simulink model "w2p4"  (R2020b)
settings: Solver=VariableStepAuto  StartTime=0.0  StopTime=10.0  RelTol=1e-3
model workspace (MAT data in the model file):
  J = Simulink.Parameter
  J.Value = 0.01
  J.DataType = 'auto'
  J.Dimensions = [1 1]
  K = Simulink.Parameter
  K.Value = 0.01
  K.DataType = 'auto'
  K.Dimensions = [1 1]
  Kd = Simulink.Parameter
  Kd.Value = 10
  Kd.DataType = 'auto'
  Kd.Dimensions = [1 1]
  Ki = Simulink.Parameter
  Ki.Value = 350
  Ki.DataType = 'auto'
  Ki.Dimensions = [1 1]
  Kp = 300
  L = Simulink.Parameter
  L.Value = 0.5
  L.DataType = 'auto'
  L.Dimensions = [1 1]
  R = Simulink.Parameter
  R.Value = 1
  R.DataType = 'auto'
  R.Dimensions = [1 1]
  b = 0.1
settings Model: Creator=Dell  LastModifiedBy=Dell

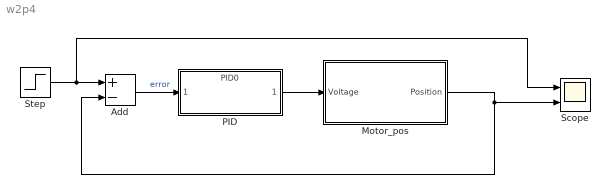
== system w2p4 ==
  Add : Sum  Inputs=+-
  Motor_pos : Subsystem
  PID : ModelReference  ModelNameDialog=PID0  SimulationMode=Normal  ModelReferenceVersion=1.3
  Scope : Scope  NumInputPorts=2
  Step : Step  SampleTime=0
  wires:
  Motor_pos/1(Position) -> Add/2, Scope/2
  PID/1 -> Motor_pos/1(Voltage)
  Step/1 -> Scope/1, Add/1
  Add/1 -> PID/1  "error"

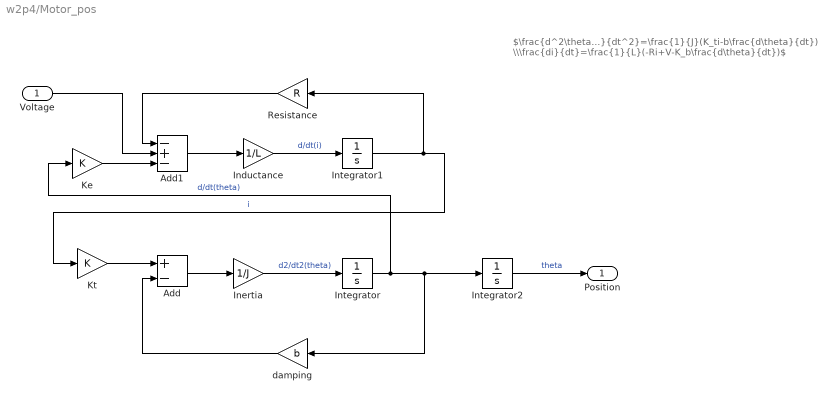
== system w2p4/Motor_pos ==
  note: $\frac{d^2\theta}{dt^2}=\frac{1}{J}(K_ti-b\frac{d\theta}{dt}) \\\frac{di}{dt}=\frac{1}{L}(-Ri+V-K_b\frac{d\theta}{dt})$
  Voltage : Inport
  Add : Sum  Inputs=+-
  Add1 : Sum  Inputs=-+-
  Inductance : Gain  Gain=1/L
  Inertia : Gain  Gain=1/J
  Integrator : Integrator
  Integrator1 : Integrator
  Integrator2 : Integrator
  Ke : Gain  Gain=K
  Kt : Gain  Gain=K
  Resistance : Gain  Gain=R
  damping : Gain  Gain=b
  Position : Outport
  wires:
  damping/1 -> Add/2
  Resistance/1 -> Add1/1
  Kt/1 -> Add/1
  Inductance/1 -> Integrator1/1  "d/dt(i)"
  Integrator1/1 -> Resistance/1, Kt/1  "i"
  Add1/1 -> Inductance/1
  Integrator2/1 -> Position/1  "theta"
  Integrator/1 -> Ke/1, damping/1, Integrator2/1  "d/dt(theta)"
  Add/1 -> Inertia/1
  Inertia/1 -> Integrator/1  "d2/dt2(theta)"
  Ke/1 -> Add1/3
  Voltage/1 -> Add1/2
